simulink model "RC_top_ACU_1"  (R2018b)
settings: Solver=VariableStepAuto  StartTime=0.0  StopTime=10000.0  RelTol=1e-3
settings Model: Creator=user  LastModifiedBy=user

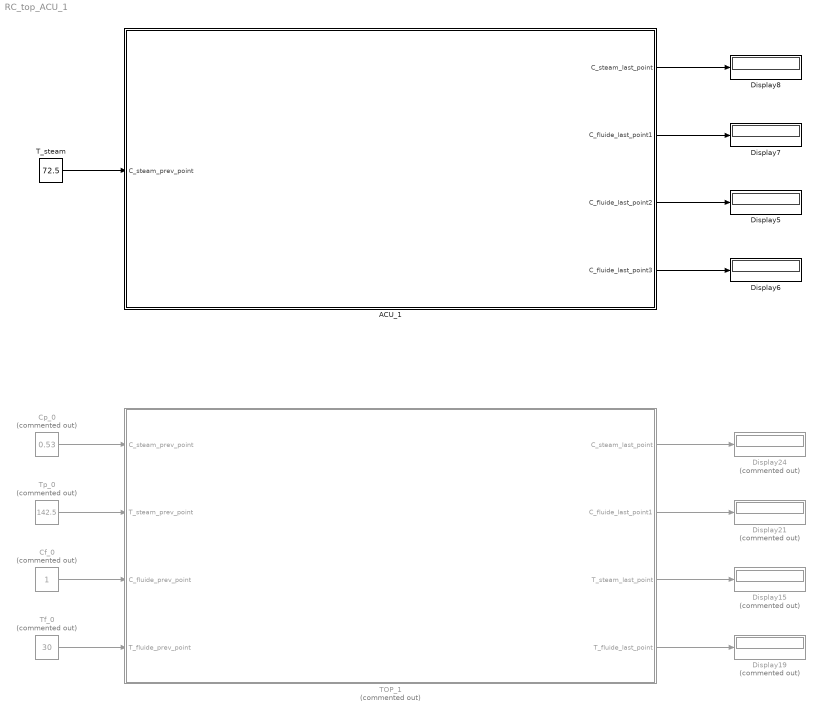
== system RC_top_ACU_1 ==
  ACU_1 : Subsystem
  Cf_0 : Constant  Commented=on
  Cp_0 : Constant  Commented=on  Value=0.53
  Display{15,19,21,24} (4 alike) : Display  Commented=on
  Display{5..8} (4 alike) : Display
  TOP_1 : Subsystem  Commented=on
  T_steam : Constant  Value=72.5
  Tf_0 : Constant  Commented=on  Value=30
  Tp_0 : Constant  Commented=on  Value=142.5
  wires:
  TOP_1/2(C_fluide_last_point1) -> Display21/1
  Tp_0/1 -> TOP_1/2(T_steam_prev_point)
  TOP_1/1(C_steam_last_point) -> Display24/1
  Cp_0/1 -> TOP_1/1(C_steam_prev_point)
  Tf_0/1 -> TOP_1/4(T_fluide_prev_point)
  TOP_1/4(T_fluide_last_point) -> Display19/1
  Cf_0/1 -> TOP_1/3(C_fluide_prev_point)
  TOP_1/3(T_steam_last_point) -> Display15/1
  T_steam/1 -> ACU_1/1(C_steam_prev_point)
  ACU_1/3(C_fluide_last_point2) -> Display5/1
  ACU_1/1(C_steam_last_point) -> Display8/1
  ACU_1/2(C_fluide_last_point1) -> Display7/1
  ACU_1/4(C_fluide_last_point3) -> Display6/1

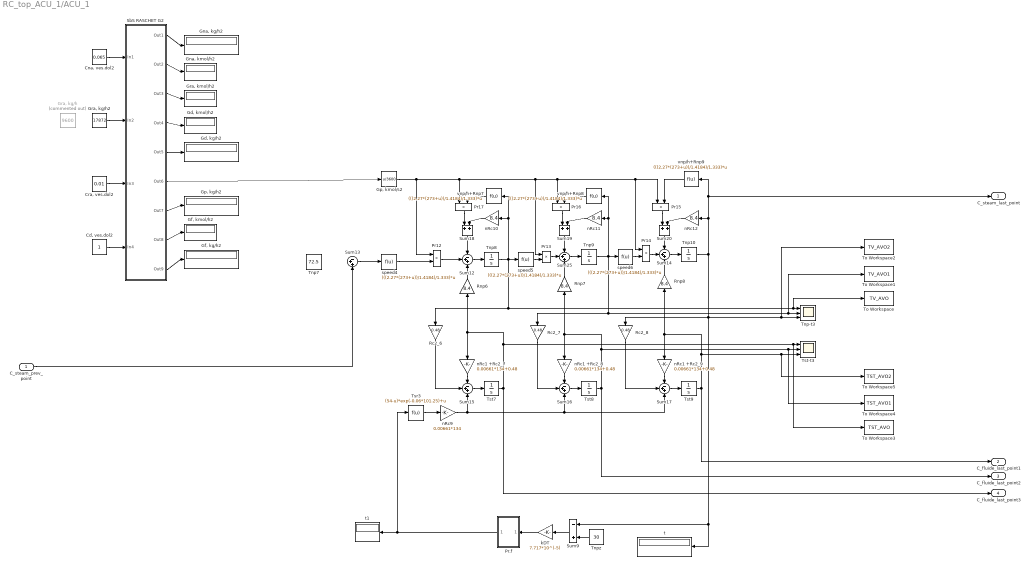
== system RC_top_ACU_1/ACU_1 ==
  C_steam_prev_point : Inport
  "Cd, ves.dol2" : Constant
  "Cna, ves.dol2" : Constant  Value=0.065
  "Cra, ves.dol2" : Constant  Value=0.01
  "Gd, kg/h2" : Display
  "Gd, kmol/h2" : Display
  "Gf, kg/h2" : Display
  "Gf, kmol/h2" : Display
  "Gna, kg/h2" : Display
  "Gna, kmol/h2" : Display
  "Gp, kmol/s2" : Fcn  Expr=u/3600
  "Gp, kg/h2" : Display
  "Gra, kg/h" : Constant  Commented=on  Value=9600
  "Gra, kg/h2" : Constant  Value=17872
  "Gra, kmol/h2" : Display
  Pr.f : Subsystem
  Pr{12..17} (6 alike) : Product  RndMeth=Zero
  Rc2_6 : Gain  Gain=0.48
  Rc2_7 : Gain  Gain=0.48
  Rc2_8 : Gain  Gain=0.48
  Rnp6 : Gain  Gain=8.4
  Rnp7 : Gain  Gain=8.4
  Rnp8 : Gain  Gain=8.4
  SbS RASCHET G2 : Subsystem
  Sum{12..17,25} (7 alike) : Sum  Inputs=-++
  Sum18 : Sum
  Sum19 : Sum
  Sum20 : Sum
  Sum9 : Sum  Inputs=-+
  Tnp-t3 : Scope  NumInputPorts=3
  Tnp10 : Integrator  InitialCondition=49.99550000
  Tnp7 : Constant  Value=72.5
  Tnp8 : Integrator  InitialCondition=64.99850000
  Tnp9 : Integrator  InitialCondition=57.49700000
  Tnpz : Constant  Value=30
  To Workspace : ToWorkspace  VariableName=TV_AVO  SaveFormat=Structure With Time  SampleTime=-1
  To Workspace1 : ToWorkspace  VariableName=TV_AVO1  SaveFormat=Structure With Time  SampleTime=-1
  To Workspace2 : ToWorkspace  VariableName=TV_AVO2  SaveFormat=Structure With Time  SampleTime=-1
  To Workspace3 : ToWorkspace  VariableName=TST_AVO  SaveFormat=Structure With Time  SampleTime=-1
  To Workspace4 : ToWorkspace  VariableName=TST_AVO1  SaveFormat=Structure With Time  SampleTime=-1
  To Workspace5 : ToWorkspace  VariableName=TST_AVO2  SaveFormat=Structure With Time  SampleTime=-1
  Tsr3 : Fcn  Expr=(54-u)*exp(-0.06*101.25)+u
  Tst-t3 : Scope  NumInputPorts=3
  Tst7 : Integrator  InitialCondition=30.749212884999000
  Tst8 : Integrator  InitialCondition=26.338794670104530
  Tst9 : Integrator  InitialCondition=23.289742144317184
  kDT : Gain  Gain=7.717*10^(-5)
  nRc1 +Rc2_7 : Gain  Gain=0.00661*134+0.48
  nRc1 +Rc2_8 : Gain  Gain=0.00661*134+0.48
  nRc1 +Rc2_9 : Gain  Gain=0.00661*134+0.48
  nRc10 : Gain  Gain=8.4
  nRc11 : Gain  Gain=8.4
  nRc12 : Gain  Gain=8.4
  nRc9 : Gain  Gain=0.00661*134
  speed4 : Fcn  Expr=(((2.27*(273+u))/1.4184)/1.333)*u
  speed5 : Fcn  Expr=(((2.27*(273+u))/1.4184)/1.333)*u
  speed6 : Fcn  Expr=(((2.27*(273+u))/1.4184)/1.333)*u
  t : Display
  t1 : Display
  vnp/h+Rnp7 : Fcn  Expr=(((2.27*(273+u))/1.4184)/1.333)*u
  vnp/h+Rnp8 : Fcn  Expr=(((2.27*(273+u))/1.4184)/1.333)*u
  vnp/h+Rnp9 : Fcn  Expr=(((2.27*(273+u))/1.4184)/1.333)*u
  C_steam_last_point : Outport
  C_fluide_last_point1 : Outport  Port=2
  C_fluide_last_point2 : Outport  Port=3
  C_fluide_last_point3 : Outport  Port=4
  wires:
  nRc1 +Rc2_7/1 -> Sum15/1
  Pr12/1 -> Sum12/2
  Sum12/1 -> Tnp8/1
  nRc1 +Rc2_9/1 -> Sum17/1
  Rc2_6/1 -> Sum15/2
  "Gra, kg/h2"/1 -> SbS RASCHET G2/2(In2)
  Pr14/1 -> Sum14/2
  SbS RASCHET G2/9(Out9) -> "Gf, kg/h2"/1
  nRc11/1 -> Sum19/2
  "Cra, ves.dol2"/1 -> SbS RASCHET G2/3(In3)
  vnp/h+Rnp8/1 -> Pr16/2
  nRc10/1 -> Sum18/2
  nRc1 +Rc2_8/1 -> Sum16/1
  Sum16/1 -> Tst8/1
  speed6/1 -> Pr14/2
  SbS RASCHET G2/7(Out7) -> "Gp, kg/h2"/1
  Rnp8/1 -> Sum14/3
  "Cna, ves.dol2"/1 -> SbS RASCHET G2/1(In1)
  Pr13/1 -> Sum25/2
  Tnp10/1 -> C_steam_last_point/1, vnp/h+Rnp9/1, nRc12/1, Sum9/1, t/1, To Workspace2/1, Tnp-t3/3, Rc2_8/1
  SbS RASCHET G2/2(Out2) -> "Gna, kmol/h2"/1
  Pr15/1 -> Sum20/1
  Tst8/1 -> C_fluide_last_point2/1, nRc1 +Rc2_8/1, Rnp7/1, To Workspace4/1, Tst-t3/2
  Sum18/1 -> Sum12/1
  Pr17/1 -> Sum18/1
  Sum19/1 -> Sum25/1
  SbS RASCHET G2/5(Out5) -> "Gd, kg/h2"/1
  Rnp7/1 -> Sum25/3
  Sum13/1 -> speed4/1
  speed4/1 -> Pr12/2
  Tsr3/1 -> nRc9/1
  "Cd, ves.dol2"/1 -> SbS RASCHET G2/4(In4)
  Sum14/1 -> Tnp10/1
  Sum25/1 -> Tnp9/1
  Rc2_8/1 -> Sum17/2
  Sum20/1 -> Sum14/1
  Rnp6/1 -> Sum12/3
  SbS RASCHET G2/8(Out8) -> "Gf, kmol/h2"/1
  SbS RASCHET G2/4(Out4) -> "Gd, kmol/h2"/1
  "Gp, kmol/s2"/1 -> Pr15/1, Pr14/1, Pr16/1, Pr13/1, Pr17/1, Pr12/1
  SbS RASCHET G2/3(Out3) -> "Gra, kmol/h2"/1
  vnp/h+Rnp9/1 -> Pr15/2
  SbS RASCHET G2/1(Out1) -> "Gna, kg/h2"/1
  Sum17/1 -> Tst9/1
  Tst9/1 -> C_fluide_last_point1/1, nRc1 +Rc2_9/1, Rnp8/1, To Workspace5/1, Tst-t3/3
  Tnp9/1 -> speed6/1, Rc2_7/1, To Workspace1/1, Tnp-t3/2, vnp/h+Rnp8/1, nRc11/1
  nRc9/1 -> Sum15/3, Sum16/3, Sum17/3
  speed5/1 -> Pr13/2
  Sum15/1 -> Tst7/1
  Tst7/1 -> C_fluide_last_point3/1, nRc1 +Rc2_7/1, Rnp6/1, Tst-t3/1, To Workspace3/1
  vnp/h+Rnp7/1 -> Pr17/2
  Tnp8/1 -> speed5/1, Rc2_6/1, To Workspace/1, Tnp-t3/1, vnp/h+Rnp7/1, nRc10/1
  Rc2_7/1 -> Sum16/2
  nRc12/1 -> Sum20/2
  Pr16/1 -> Sum19/1
  C_steam_prev_point/1 -> Sum13/3
  Pr.f/1(Out1) -> Tsr3/1, t1/1
  Sum9/1 -> kDT/1
  Tnpz/1 -> Sum9/2
  kDT/1 -> Pr.f/1(In1)
  SbS RASCHET G2/6(Out6) -> "Gp, kmol/s2"/1

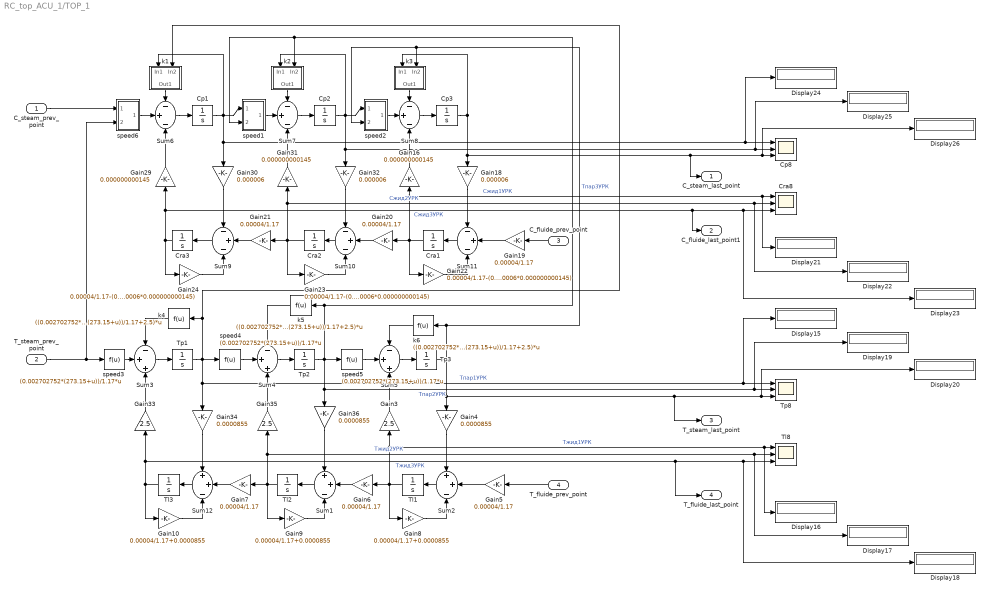
== system RC_top_ACU_1/TOP_1 ==
  C_steam_prev_point : Inport
  T_steam_prev_point : Inport  Port=2
  C_fluide_prev_point : Inport  Port=3
  T_fluide_prev_point : Inport  Port=4
  Cp1 : Integrator  InitialCondition=0.68200000
  Cp2 : Integrator  InitialCondition=0.83400000
  Cp3 : Integrator  InitialCondition=0.98600000
  Cp8 : Scope  NumInputPorts=3
  Cra1 : Integrator  InitialCondition=0.88825000
  Cra2 : Integrator  InitialCondition=0.77650000
  Cra3 : Integrator  InitialCondition=0.66475000
  Cra8 : Scope  NumInputPorts=3
  Display{15..26} (12 alike) : Display
  Gain10 : Gain  Gain=0.00004/1.17+0.0000855
  Gain16 : Gain  Gain=0.000000000145
  Gain18 : Gain  Gain=0.000006
  Gain{5..7,19..21} (6 alike) : Gain  Gain=0.00004/1.17
  Gain22 : Gain  Gain=0.00004/1.17-(0.000006*0.000000000145)
  Gain23 : Gain  Gain=0.00004/1.17-(0.000006*0.000000000145)
  Gain24 : Gain  Gain=0.00004/1.17-(0.000006*0.000000000145)
  Gain29 : Gain  Gain=0.000000000145
  Gain3 : Gain  Gain=2.5
  Gain30 : Gain  Gain=0.000006
  Gain31 : Gain  Gain=0.000000000145
  Gain32 : Gain  Gain=0.000006
  Gain33 : Gain  Gain=2.5
  Gain34 : Gain  Gain=0.0000855
  Gain35 : Gain  Gain=2.5
  Gain36 : Gain  Gain=0.0000855
  Gain4 : Gain  Gain=0.0000855
  Gain8 : Gain  Gain=0.00004/1.17+0.0000855
  Gain9 : Gain  Gain=0.00004/1.17+0.0000855
  Sum1 : Sum  Inputs=++-
  Sum{6..11} (6 alike) : Sum  Inputs=-+-
  Sum12 : Sum  Inputs=++-
  Sum2 : Sum  Inputs=++-
  Sum3 : Sum  Inputs=-++
  Sum4 : Sum  Inputs=-++
  Sum5 : Sum  Inputs=-++
  Tl1 : Integrator  InitialCondition=57.25000000
  Tl2 : Integrator  InitialCondition=84.50000000
  Tl3 : Integrator  InitialCondition=111.75000000
  Tl8 : Scope  NumInputPorts=3
  Tp1 : Integrator  InitialCondition=118.20000000
  Tp2 : Integrator  InitialCondition=93.90000000
  Tp3 : Integrator  InitialCondition=69.60000000  IgnoreLimit=on
  Tp8 : Scope  NumInputPorts=3
  k1 : Subsystem
  k2 : Subsystem
  k3 : Subsystem
  k4 : Fcn  Expr=((0.002702752*(273.15+u))/1.17+2.5)*u
  k5 : Fcn  Expr=((0.002702752*(273.15+u))/1.17+2.5)*u
  k6 : Fcn  Expr=((0.002702752*(273.15+u))/1.17+2.5)*u
  speed1 : Subsystem
  speed2 : Subsystem
  speed3 : Fcn  Expr=(0.002702752*(273.15+u))/1.17*u
  speed4 : Fcn  Expr=(0.002702752*(273.15+u))/1.17*u
  speed5 : Fcn  Expr=(0.002702752*(273.15+u))/1.17*u
  speed6 : Subsystem
  C_steam_last_point : Outport
  C_fluide_last_point1 : Outport  Port=2
  T_steam_last_point : Outport  Port=3
  T_fluide_last_point : Outport  Port=4
  wires:
  speed4/1 -> Sum4/2
  C_steam_prev_point/1 -> speed6/1(In1)
  T_fluide_prev_point/1 -> Gain5/1
  Sum4/1 -> Tp2/1
  C_fluide_prev_point/1 -> Gain19/1
  Tl1/1 -> Gain8/1, Gain6/1, Display16/1, Tl8/1, Gain3/1  "Tжид1УРК"
  Gain32/1 -> Sum10/1
  Sum6/1 -> Cp1/1
  k3/1(Out1) -> Sum8/1
  k4/1 -> Sum3/1
  Gain24/1 -> Sum9/3
  Gain10/1 -> Sum12/3
  speed3/1 -> Sum3/2
  Gain29/1 -> Sum6/3
  Sum9/1 -> Cra3/1
  Sum11/1 -> Cra1/1
  Gain21/1 -> Sum9/2
  Cp2/1 -> Display25/1, Cp8/2, Gain32/1, speed2/1(In1), k2/1(In1)
  speed6/1(Out1) -> Sum6/2
  Cp1/1 -> Cp8/1, Display24/1, Gain30/1, k1/1(In1), speed1/1(In1)
  Gain3/1 -> Sum5/3
  Tl2/1 -> Gain9/1, Gain7/1, Display17/1, Tl8/2, Gain35/1  "Tжид2УРК"
  Gain31/1 -> Sum7/3
  Cra3/1 -> Gain24/1, C_fluide_last_point1/1, Display23/1, Cra8/3, Gain29/1  "Cжид3УРК"
  Cp3/1 -> C_steam_last_point/1, Display26/1, Cp8/3, Gain18/1, k3/1(In1)
  Sum10/1 -> Cra2/1
  Tp1/1 -> Display15/1, Tp8/1, Gain34/1, k4/1, k1/2(In2), speed4/1  "Tпар1УРК"
  Cra1/1 -> Gain22/1, Gain20/1, Display21/1, Cra8/1, Gain16/1  "Cжид1УРК"
  Sum7/1 -> Cp2/1
  Gain23/1 -> Sum10/3
  Gain8/1 -> Sum2/3
  Gain30/1 -> Sum9/1
  k2/1(Out1) -> Sum7/1
  Gain34/1 -> Sum12/1
  Sum12/1 -> Tl3/1
  Tp3/1 -> T_steam_last_point/1, Display20/1, Tp8/3, Gain4/1, k6/1, k3/2(In2), speed2/2(In2)  "Tпар3УРК"
  Gain20/1 -> Sum10/2
  k6/1 -> Sum5/1
  Sum2/1 -> Tl1/1
  k5/1 -> Sum4/1
  Sum1/1 -> Tl2/1
  Tp2/1 -> Display19/1, Tp8/2, Gain36/1, k5/1, k2/2(In2), speed1/2(In2), speed5/1  "Tпар2УРК"
  Gain4/1 -> Sum2/1
  Sum3/1 -> Tp1/1
  Gain6/1 -> Sum1/2
  Gain18/1 -> Sum11/1
  Tl3/1 -> Gain10/1, T_fluide_last_point/1, Display18/1, Tl8/3, Gain33/1  "Tжид3УРК"
  Gain9/1 -> Sum1/3
  k1/1(Out1) -> Sum6/1
  Gain19/1 -> Sum11/2
  Gain7/1 -> Sum12/2
  speed2/1(Out1) -> Sum8/2
  Sum5/1 -> Tp3/1
  Gain35/1 -> Sum4/3
  T_steam_prev_point/1 -> speed6/2(In2), speed3/1
  Sum8/1 -> Cp3/1
  Gain22/1 -> Sum11/3
  Gain16/1 -> Sum8/3
  Gain33/1 -> Sum3/3
  Gain5/1 -> Sum2/2
  speed5/1 -> Sum5/2
  Cra2/1 -> Gain23/1, Gain21/1, Display22/1, Cra8/2, Gain31/1  "Cжид2УРК"
  speed1/1(Out1) -> Sum7/2
  Gain36/1 -> Sum1/1

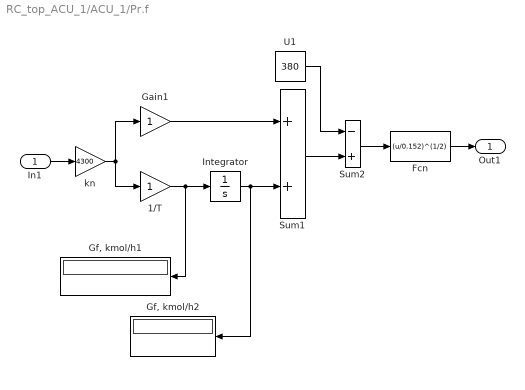
== system RC_top_ACU_1/ACU_1/Pr.f ==
  In1 : Inport
  1/T : Gain
  Fcn : Fcn  Expr=(u/0.152)^(1/2)
  Gain1 : Gain
  "Gf, kmol/h1" : Display
  "Gf, kmol/h2" : Display
  Integrator : Integrator  InitialCondition=403.6
  Sum1 : Sum
  Sum2 : Sum  Inputs=-+
  U1 : Constant  Value=380
  kn : Gain  Gain=4300
  Out1 : Outport
  wires:
  kn/1 -> 1/T/1, Gain1/1
  1/T/1 -> Integrator/1, "Gf, kmol/h1"/1
  Integrator/1 -> Sum1/2, "Gf, kmol/h2"/1
  Gain1/1 -> Sum1/1
  Sum1/1 -> Sum2/2
  U1/1 -> Sum2/1
  In1/1 -> kn/1
  Fcn/1 -> Out1/1
  Sum2/1 -> Fcn/1

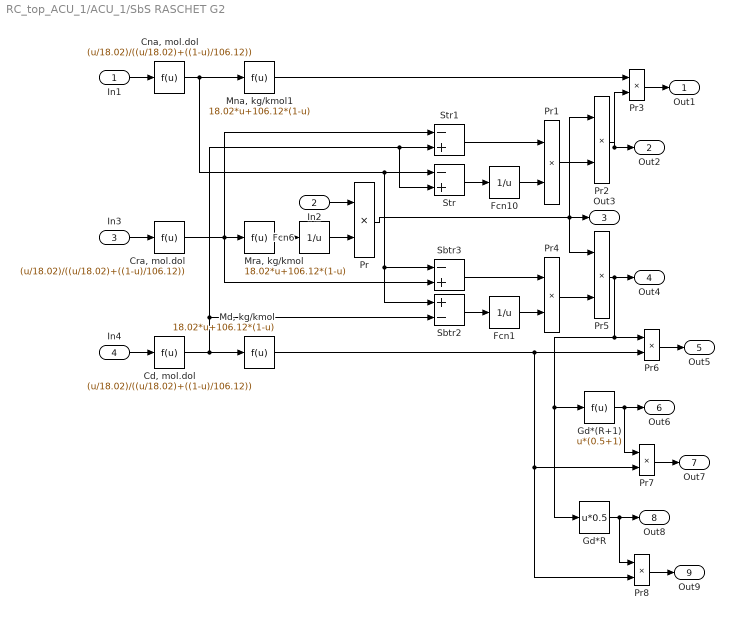
== system RC_top_ACU_1/ACU_1/SbS RASCHET G2 ==
  In1 : Inport
  In2 : Inport  Port=2
  In3 : Inport  Port=3
  In4 : Inport  Port=4
  "Cd, mol.dol" : Fcn  Expr=(u/18.02)/((u/18.02)+((1-u)/106.12))
  "Cna, mol.dol" : Fcn  Expr=(u/18.02)/((u/18.02)+((1-u)/106.12))
  "Cra, mol.dol" : Fcn  Expr=(u/18.02)/((u/18.02)+((1-u)/106.12))
  Fcn1 : Fcn  Expr=1/u
  Fcn10 : Fcn  Expr=1/u
  Fcn6 : Fcn  Expr=1/u
  Gd*(R+1) : Fcn  Expr=u*(0.5+1)
  Gd*R : Fcn  Expr=u*0.5
  "Md, kg/kmol" : Fcn  Expr=18.02*u+106.12*(1-u)
  "Mna, kg/kmol1" : Fcn  Expr=18.02*u+106.12*(1-u)
  "Mra, kg/kmol" : Fcn  Expr=18.02*u+106.12*(1-u)
  Pr{,1..8} (9 alike) : Product  RndMeth=Zero
  Sbtr2 : Sum  Inputs=+-
  Sbtr3 : Sum  Inputs=-+
  Str : Sum  Inputs=-+
  Str1 : Sum  Inputs=-+
  Out1 : Outport
  Out2 : Outport  Port=2
  Out3 : Outport  Port=3
  Out4 : Outport  Port=4
  Out5 : Outport  Port=5
  Out6 : Outport  Port=6
  Out7 : Outport  Port=7
  Out8 : Outport  Port=8
  Out9 : Outport  Port=9
  wires:
  "Mna, kg/kmol1"/1 -> Pr3/1
  "Cna, mol.dol"/1 -> "Mna, kg/kmol1"/1, Str/1, Sbtr3/1, Sbtr2/1
  "Cra, mol.dol"/1 -> "Mra, kg/kmol"/1, Str1/1, Sbtr3/2
  "Cd, mol.dol"/1 -> "Md, kg/kmol"/1, Str1/2, Str/2, Sbtr2/2
  "Mra, kg/kmol"/1 -> Fcn6/1
  Fcn6/1 -> Pr/2
  Pr/1 -> Pr2/1, Out3/1, Pr5/1
  Str/1 -> Fcn10/1
  Fcn10/1 -> Pr1/2
  Pr2/1 -> Pr3/2, Out2/1
  Pr1/1 -> Pr2/2
  Str1/1 -> Pr1/1
  Fcn1/1 -> Pr4/2
  Pr5/1 -> Pr6/1, Gd*(R+1)/1, Gd*R/1, Out4/1
  Pr4/1 -> Pr5/2
  "Md, kg/kmol"/1 -> Pr6/2, Pr7/2, Pr8/2
  Sbtr2/1 -> Fcn1/1
  Sbtr3/1 -> Pr4/1
  Gd*(R+1)/1 -> Pr7/1, Out6/1
  Gd*R/1 -> Pr8/1, Out8/1
  In1/1 -> "Cna, mol.dol"/1
  Pr3/1 -> Out1/1
  In2/1 -> Pr/1
  In3/1 -> "Cra, mol.dol"/1
  Pr6/1 -> Out5/1
  In4/1 -> "Cd, mol.dol"/1
  Pr7/1 -> Out7/1
  Pr8/1 -> Out9/1

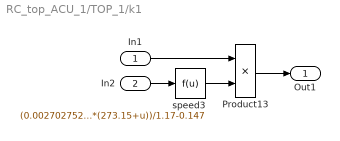
== system RC_top_ACU_1/TOP_1/k1 ==
  In1 : Inport
  In2 : Inport  Port=2
  Product13 : Product  SaturateOnIntegerOverflow=on  InputSameDT=on  OutDataTypeStr=Inherit: Same as first input
  speed3 : Fcn  Expr=(0.002702752*(273.15+u))/1.17-0.147
  Out1 : Outport
  wires:
  Product13/1 -> Out1/1
  speed3/1 -> Product13/2
  In2/1 -> speed3/1
  In1/1 -> Product13/1

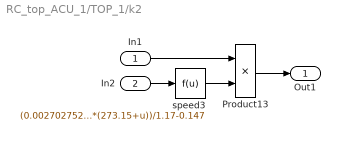
== system RC_top_ACU_1/TOP_1/k2 ==
  In1 : Inport
  In2 : Inport  Port=2
  Product13 : Product  SaturateOnIntegerOverflow=on  InputSameDT=on  OutDataTypeStr=Inherit: Same as first input
  speed3 : Fcn  Expr=(0.002702752*(273.15+u))/1.17-0.147
  Out1 : Outport
  wires:
  In1/1 -> Product13/1
  In2/1 -> speed3/1
  speed3/1 -> Product13/2
  Product13/1 -> Out1/1

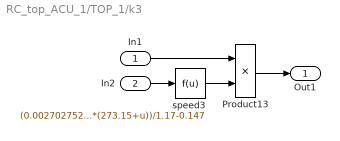
== system RC_top_ACU_1/TOP_1/k3 ==
  In1 : Inport
  In2 : Inport  Port=2
  Product13 : Product  SaturateOnIntegerOverflow=on  InputSameDT=on  OutDataTypeStr=Inherit: Same as first input
  speed3 : Fcn  Expr=(0.002702752*(273.15+u))/1.17-0.147
  Out1 : Outport
  wires:
  Product13/1 -> Out1/1
  speed3/1 -> Product13/2
  In2/1 -> speed3/1
  In1/1 -> Product13/1

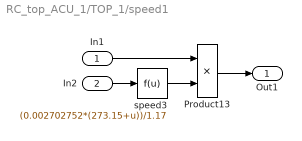
== system RC_top_ACU_1/TOP_1/speed1 ==
  In1 : Inport
  In2 : Inport  Port=2
  Product13 : Product  SaturateOnIntegerOverflow=on  InputSameDT=on  OutDataTypeStr=Inherit: Same as first input
  speed3 : Fcn  Expr=(0.002702752*(273.15+u))/1.17
  Out1 : Outport
  wires:
  Product13/1 -> Out1/1
  speed3/1 -> Product13/2
  In2/1 -> speed3/1
  In1/1 -> Product13/1

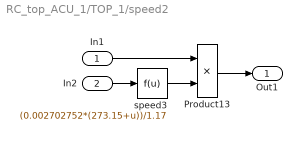
== system RC_top_ACU_1/TOP_1/speed2 ==
  In1 : Inport
  In2 : Inport  Port=2
  Product13 : Product  SaturateOnIntegerOverflow=on  InputSameDT=on  OutDataTypeStr=Inherit: Same as first input
  speed3 : Fcn  Expr=(0.002702752*(273.15+u))/1.17
  Out1 : Outport
  wires:
  In1/1 -> Product13/1
  In2/1 -> speed3/1
  speed3/1 -> Product13/2
  Product13/1 -> Out1/1

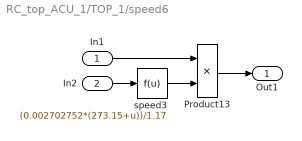
== system RC_top_ACU_1/TOP_1/speed6 ==
  In1 : Inport
  In2 : Inport  Port=2
  Product13 : Product  SaturateOnIntegerOverflow=on  InputSameDT=on  OutDataTypeStr=Inherit: Same as first input
  speed3 : Fcn  Expr=(0.002702752*(273.15+u))/1.17
  Out1 : Outport
  wires:
  In1/1 -> Product13/1
  In2/1 -> speed3/1
  speed3/1 -> Product13/2
  Product13/1 -> Out1/1
